simulink model "monofasikos_ask5.1_monofasikos"  (R2021a)
settings: Solver=ode23tb  StartTime=0.0  StopTime=56  MaxStep=1e-5  RelTol=1e-3
libraries: spsRMSLib x4, spsCurrentMeasurementLib x2, spsSaturableTransformerLib x2, spsVoltageMeasurementLib x2, spsControlledVoltageSourceLib x1, simulink x1, spsPowerLib x1, spsSeriesRLCBranchLib x1, spsDCVoltageSourceLib x1, spspowerguiLib x1
settings Model: Creator=User  LastModifiedBy=epape
settings SolverCC: AlgebraicLoopSolver=TrustRegion
settings DebuggingCC: SFMachineParentedDataDiag=warning

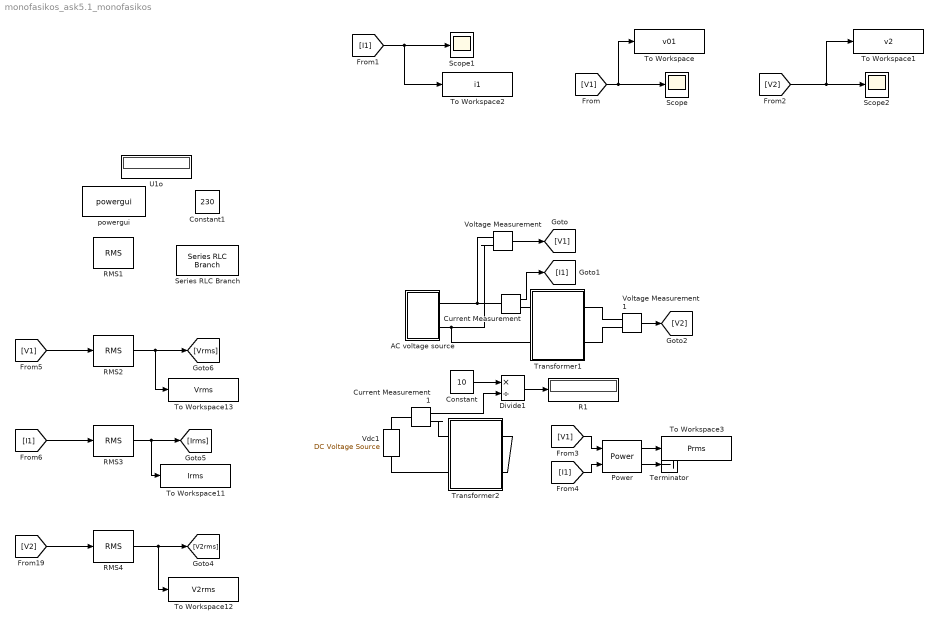
== system monofasikos_ask5.1_monofasikos ==
  AC voltage source : Subsystem  mask{Vrms=230}
  Constant : Constant  Value=10
  Constant1 : Constant  Value=230
  Current Measurement : spsCurrentMeasurementLib/Current Measurement  PhasorSimulation=off  OutputType=Complex  PSBequivalent=0
  Current Measurement1 : spsCurrentMeasurementLib/Current Measurement  PhasorSimulation=off  OutputType=Complex  PSBequivalent=0
  Divide1 : Product  Inputs=*/
  Power : spsPowerLib/Power  Freq=50  Vinit=[0, 0]  Iinit=[0, 0]  Ts=1e-5
      settings: SourceProductBaseCode=PS
  R1 : Display
  RMS{1..4} (4 alike) : spsRMSLib/RMS  TrueRMS=on  Freq=50  RMSInit=0  Ts=0
  Scope : Scope
  Scope1 : Scope
  Scope2 : Scope
  Series RLC Branch : spsSeriesRLCBranchLib/Series RLC Branch  LConnTagsString=__new0  RConnTagsString=__new0  BranchType=RLC  Resistance=1  Inductance=1e-3  SetiL0=off  InitialCurrent=0  Capacitance=1e-6  Setx0=off  InitialVoltage=0  Measurements=None
  Terminator : Terminator
  To Workspace : ToWorkspace  VariableName=v01  SaveFormat=Timeseries  SampleTime=1e-5
  To Workspace1 : ToWorkspace  VariableName=v2  SaveFormat=Timeseries  SampleTime=1e-5
  To Workspace11 : ToWorkspace  VariableName=Irms  SaveFormat=Timeseries  SampleTime=1e-5
  To Workspace12 : ToWorkspace  VariableName=V2rms  SaveFormat=Timeseries  SampleTime=1e-5
  To Workspace13 : ToWorkspace  VariableName=Vrms  SaveFormat=Timeseries  SampleTime=1e-5
  To Workspace2 : ToWorkspace  VariableName=i1  SaveFormat=Timeseries  SampleTime=1e-5
  To Workspace3 : ToWorkspace  VariableName=Prms  SaveFormat=Timeseries  SampleTime=1e-5
  Transformer1 : Subsystem  mask{PN=4, U1N=230, U2N=115}
      mask prompts: PN "PN (kVA)"; U1N "U1N (V)"; U2N "U2N (V)"
  Transformer2 : Subsystem  mask{PN=4, U1N=230, U2N=115}
      mask prompts: PN "PN (kVA)"; U1N "U1N (V)"; U2N "U2N (V)"
  U1o : Display
  Vdc1 : spsDCVoltageSourceLib/DC Voltage Source  Amplitude=10  Measurements=Voltage
  Voltage Measurement : spsVoltageMeasurementLib/Voltage Measurement  PhasorSimulation=off  OutputType=Complex  PSBequivalent=0
  Voltage Measurement1 : spsVoltageMeasurementLib/Voltage Measurement  PhasorSimulation=off  OutputType=Complex  PSBequivalent=0
  powergui : spspowerguiLib/powergui  Priority=1  SimulationMode=Continuous  SampleTime=50e-6  frequency=60  Iterations=50  frequencyindice=0  Pbase=100e6  ErrMax=1e-4  UnitsV=kV  UnitsW=MW  buscounter=0  FunctionMessages=off  echomessages=off  EnableUseOfTLC=off  CurrentSourceSwitches=off  DisableSnubberDevices=off  DisableRonSwitches=off  DisableVfSwitches=off  DisplayEquations=off  AutomaticDiscreteSolvers=off  SolverType=Tustin/Backward Euler (TBE)  Interpol=off  ExternalGateDelay=off  methode=off  Ts=100  x0status=blocks  SPID=on  SwTol=0  HookPort=off  NonlinearTolerance=1e-4  nMaxIteration=100  ContinueOnMaxIteration=off  RestoreLinks=warning  ResistiveCurrentMeasurement=off  Frange=[0:2:500]  Ylog=off  Xlog=on  ShowGrid=off  save=off  variable=ZData  structure=0  ZoomFFT=off  StartTime=0.0  cycles=1  DisplayStyle=1  fundamental=60  FreqAxis=off  MaxFrequency=1000  frequencyindicesteady=1  RmsSteady=1  display=off
  wires:
  Voltage Measurement/1 -> [V1]
  Current Measurement/1 -> [I1]
  Voltage Measurement1/1 -> [V2]
  [V1] -> To Workspace/1, Scope/1
  [I1] -> To Workspace2/1, Scope1/1
  [V2] -> To Workspace1/1, Scope2/1
  [V1] -> Power/1
  [I1] -> Power/2
  Power/1 -> To Workspace3/1
  [V1] -> RMS2/1
  [I1] -> RMS3/1
  RMS2/1 -> To Workspace13/1, [Vrms]
  RMS3/1 -> To Workspace11/1, [Irms]
  Current Measurement1/1 -> Divide1/2
  Constant/1 -> Divide1/1
  Divide1/1 -> R1/1
  RMS4/1 -> To Workspace12/1, [V2rms]
  [V2] -> RMS4/1
  Power/2 -> Terminator/1
  connections:
  AC voltage source/RConn1 -- Voltage Measurement/LConn1 -- Current Measurement/LConn1
  AC voltage source/RConn2 -- Transformer1/LConn2 -- Voltage Measurement/LConn2
  Transformer1/RConn1 -- Voltage Measurement1/LConn1
  Transformer1/RConn2 -- Voltage Measurement1/LConn2
  Vdc1/LConn1 -- Transformer2/LConn2
  Transformer1/LConn1 -- Current Measurement/RConn1
  Vdc1/RConn1 -- Current Measurement1/LConn1
  Current Measurement1/RConn1 -- Transformer2/LConn1
  Transformer2/RConn1 -- Transformer2/RConn2

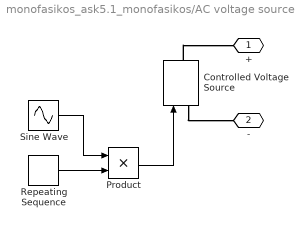
== system monofasikos_ask5.1_monofasikos/AC voltage source ==
  Controlled Voltage Source : spsControlledVoltageSourceLib/Controlled Voltage Source  Initialize=on  Source_Type=AC  Amplitude=0  Phase=0  Frequency=50  Measurements=Voltage
  Product : Product
  Repeating Sequence : simulink/Sources/Repeating Sequence  rep_seq_t=t  rep_seq_y=Vs
  Sine Wave : Sin  Amplitude=sqrt(2)  Frequency=100*pi  SampleTime=0
  + : PMIOPort  Side=Right
  - : PMIOPort  Port=2  Side=Right
  wires:
  Product/1 -> Controlled Voltage Source/1
  Sine Wave/1 -> Product/1
  Repeating Sequence/1 -> Product/2
  connections:
  Controlled Voltage Source/LConn1 -- -/RConn1
  Controlled Voltage Source/RConn1 -- +/RConn1

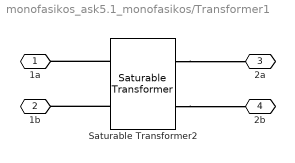
== system monofasikos_ask5.1_monofasikos/Transformer1 ==
  Saturable Transformer2 : spsSaturableTransformerLib/Saturable Transformer  ThreeWindings=off  Hysteresis=off  DataFile='hysteresis.mat'  Measurements=None  UNITS=pu  NominalPower=[4e3 50]  Winding1=[230 0.022273 0.015903]  Winding2=[122 0.024298 0.019083]  Winding3=[3.15e+05 0.00245 0.098001]  Saturation=[0 0;0.031714 0.76205;0.037813 0.86926;0.045538 0.94653;0.060175 1.0141;0.080911 1.0624;0.14637 1.159]  CoreLoss=35.539  BreakLoop=off  DiscreteSolver=Trapezoidal iterative  DataType=off  InitialFlux=0  TransfoNumber=1
      settings: SourceProductBaseCode=PS
  1a : PMIOPort  Side=Left
  1b : PMIOPort  Port=2  Side=Left
  2a : PMIOPort  Port=3  Side=Right
  2b : PMIOPort  Port=4  Side=Right
  connections:
  Saturable Transformer2/RConn2 -- 2b/RConn1
  Saturable Transformer2/LConn1 -- 1a/RConn1
  Saturable Transformer2/RConn1 -- 2a/RConn1
  Saturable Transformer2/LConn2 -- 1b/RConn1

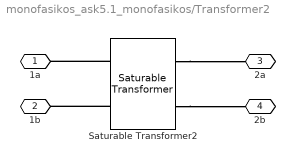
== system monofasikos_ask5.1_monofasikos/Transformer2 ==
  Saturable Transformer2 : spsSaturableTransformerLib/Saturable Transformer  ThreeWindings=off  Hysteresis=off  DataFile='hysteresis.mat'  Measurements=None  UNITS=SI  NominalPower=[4e3 50]  Winding1=[230 0.29456 0.00066946]  Winding2=[122 0.090413 0.00022602]  Winding3=[3.15e+05 60775 7738.2]  Saturation=[0 0;0.78001 0.789;0.93001 0.9;1.12 0.98;1.48 1.05;1.99 1.1;3.6 1.2]  CoreLoss=470  BreakLoop=off  DiscreteSolver=Trapezoidal iterative  DataType=on  InitialFlux=0  TransfoNumber=1
      settings: SourceProductBaseCode=PS
  1a : PMIOPort  Side=Left
  1b : PMIOPort  Port=2  Side=Left
  2a : PMIOPort  Port=3  Side=Right
  2b : PMIOPort  Port=4  Side=Right
  connections:
  Saturable Transformer2/RConn2 -- 2b/RConn1
  Saturable Transformer2/LConn1 -- 1a/RConn1
  Saturable Transformer2/RConn1 -- 2a/RConn1
  Saturable Transformer2/LConn2 -- 1b/RConn1
